simulink model "cantoni_combined_matrices_3pools_gates_hil_test"  (R2019b)
settings: Solver=FixedStepDiscrete  StartTime=0.0  StopTime=1000  FixedStep=1  RelTol=1e-3
values from neighbouring files (symbols this model uses):
  comb_contr = ss(Ac, Bc, Cc, Dc, h)    [cantoni_LMI.m]
  comb_plant_disc = c2d(comb_plant_cont,h,'zoh')    [cantoni_LMI.m]
  ddelay = [4 2 4 4 6]    [distributed_workspace.mat]
  Pd0 = c2d(P0, h, 'zoh')    [model_hil.m]
undefined symbols (not defined in the file or in its folder): Pd, Wd, Wis
settings Model: Creator=Jacob  LastModifiedBy=bas
settings SFSimCC: CustomCodeUndefinedFunction=UseInterfaceOnly

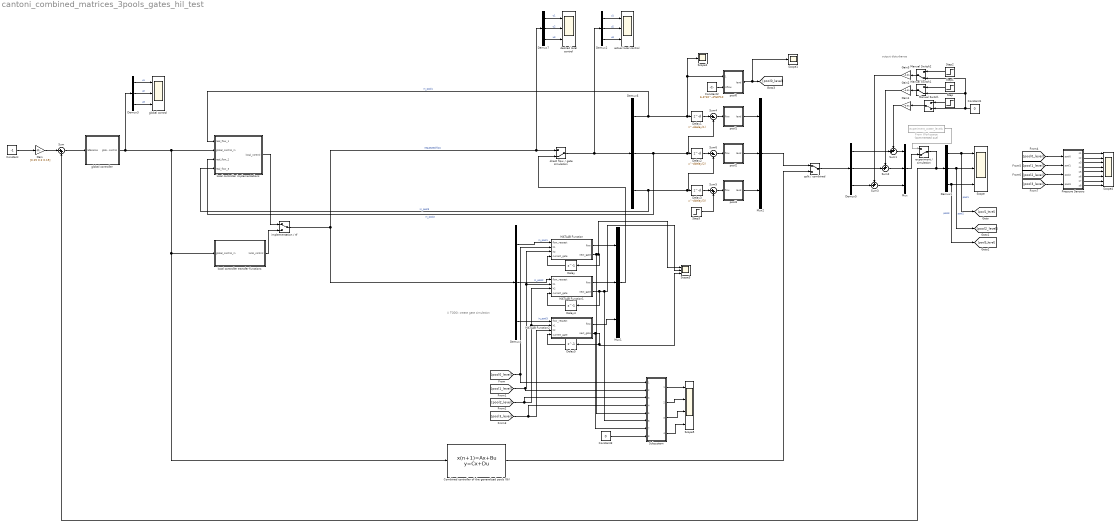
== system cantoni_combined_matrices_3pools_gates_hil_test ==
  note: // TODO: create gate simulation
  note: output disturbance
  Combined controller of the generalized pools (Gi) : DiscreteStateSpace  A=comb_plant_disc.A  B=comb_plant_disc.B  C=comb_plant_disc.C  D=comb_plant_disc.D  SampleTime=-1
  Constant : Constant  Value=-1
  Constant1 : Constant  Value=0
  Constant2 : Constant  Value=6.4*10^-4*60*10
  Constant3 : Constant  Value=0
  Delay : Delay  DelayLength=1
  Delay1 : Delay  DelayLength=ddelay(1)
  Delay2 : Delay  DelayLength=ddelay(2)
  Delay3 : Delay  DelayLength=ddelay(3)
  Delay4 : Delay  DelayLength=1
  Delay5 : Delay  DelayLength=1
  Demux{1..7} (7 alike) : Demux  Outputs=3
  From Workspace : FromWorkspace  Commented=on  VariableName=experiment_water_levels
  Gain : Gain  Gain=[0.25 0.2 0.15]
  Gain1 : Gain  Gain=-0.01
  Gain2 : Gain  Gain=-0.01
  Gain3 : Gain  Gain=-0.01
  MATLAB Function : MATLAB Function  TreatAsAtomicUnit=on
  MATLAB Function1 : MATLAB Function  TreatAsAtomicUnit=on
  MATLAB Function2 : MATLAB Function  TreatAsAtomicUnit=on
  Manual Switch : ManualSwitch  CurrentSetting=0
  Manual Switch1 : ManualSwitch  CurrentSetting=0
  Manual Switch2 : ManualSwitch  CurrentSetting=0
  Mux : Mux  Inputs=3
  Mux1 : Mux  Inputs=3
  Mux2 : Mux  Inputs=3
  Pressure Sensors : Subsystem
  Scope : Scope  NumInputPorts=3
  Scope1 : Scope
  Scope2 : Scope
  Scope3 : Scope  NumInputPorts=3
  Scope4 : Scope  NumInputPorts=8
  Scope5 : Scope  NumInputPorts=4
  Step : Step  Time=50  SampleTime=0
  Step1 : Step  Time=50  SampleTime=0
  Step2 : Step  Time=50  SampleTime=0
  Step3 : Step  Time=400  After=-3*10^-4*60*1  SampleTime=0
  Subsystem : Subsystem
  Sum : Sum  Inputs=|++
  Sum1 : Sum  Inputs=++|
  Sum2 : Sum  Inputs=++|
  Sum3 : Sum  Inputs=++|
  Sum4 : Sum  Inputs=|+-
  Sum5 : Sum  Inputs=|++
  Sum6 : Sum  Inputs=|+-
  actual local control : Scope  NumInputPorts=3
  desired local control : Scope  NumInputPorts=3
  direct flow / gate simulation : ManualSwitch  CurrentSetting=0
  experiment / simulation : ManualSwitch  CurrentSetting=0
  global control : Scope  NumInputPorts=3
  global controller : Subsystem
  implementation / tf : ManualSwitch
  local controller implementations : Subsystem
  local controller transfer functions : Subsystem
  pool0 : Subsystem
  pool1 : Subsystem
  pool2 : Subsystem
  pool3 : Subsystem
  split / combined : ManualSwitch
  wires:
  Constant/1 -> Gain/1
  Gain/1 -> Sum/1
  experiment / simulation/1 -> Sum/2, Demux1/1
  Demux1/1 -> Scope/1, [pool1_level]  "pool1"
  Demux1/2 -> [pool2_level], Scope/2  "pool2"
  Demux1/3 -> [pool3_level], Scope/3  "pool3"
  Step/1 -> Manual Switch/1
  Sum1/1 -> Mux/1
  Sum2/1 -> Mux/2
  Gain2/1 -> Sum2/1
  Step1/1 -> Manual Switch1/1
  Gain1/1 -> Sum1/1
  Manual Switch/1 -> Gain1/1
  Constant1/1 -> Manual Switch1/2, Manual Switch2/2, Manual Switch/2
  Manual Switch1/1 -> Gain2/1
  Sum3/1 -> Mux/3
  Manual Switch2/1 -> Gain3/1
  Step2/1 -> Manual Switch2/1
  Gain3/1 -> Sum3/1
  Demux3/3 -> global control/3  "u3"
  Demux3/2 -> global control/2  "u2"
  Demux3/1 -> global control/1  "u1"
  Demux5/1 -> Sum1/2
  Demux5/2 -> Sum2/2
  Demux5/3 -> Sum3/2
  split / combined/1 -> Demux5/1
  Mux2/1 -> split / combined/1
  Combined controller of the generalized pools (Gi)/1 -> split / combined/2
  Delay1/1 -> Sum4/1
  Delay2/1 -> Sum6/1
  Demux6/1 -> Scope2/1, pool0/1(outflow), Delay1/1, local controller implementations/1(real_flow_1)  "in_pool1"
  Demux6/2 -> Sum4/2, Delay2/1, local controller implementations/3(real_flow_2)  "in_pool2"
  Demux6/3 -> Sum6/2, Delay3/1, local controller implementations/4(real_flow_3)  "in_pool3"
  implementation / tf/1 -> Demux4/1, Demux7/1, direct flow / gate simulation/1  "requested flow"
  local controller implementations/1(local_control) -> implementation / tf/1
  local controller transfer functions/1(local_control) -> implementation / tf/2
  Mux1/1 -> direct flow / gate simulation/2
  Sum4/1 -> pool1/1(flow)
  pool1/1(level) -> Mux2/1
  Sum6/1 -> pool2/1(flow)
  pool2/1(level) -> Mux2/2
  Delay3/1 -> Sum5/1
  pool3/1(level) -> Mux2/3
  global controller/1(global_control) -> local controller implementations/2(global_control_in), local controller transfer functions/1(global_control_in), Combined controller of the generalized pools (Gi)/1, Demux3/1
  Sum/1 -> global controller/1(reference)
  Demux2/3 -> actual local control/3  "u3"
  Demux2/1 -> actual local control/1  "u1"
  Demux2/2 -> actual local control/2  "u2"
  direct flow / gate simulation/1 -> Demux2/1, Demux6/1
  pool0/1(level) -> Scope1/1, [pool0_level]
  MATLAB Function/1(flow) -> Mux1/1
  Demux4/1 -> MATLAB Function/1(flow_request)  "in_pool1"
  Demux4/2 -> MATLAB Function1/1(flow_request)  "in_pool2"
  Demux4/3 -> MATLAB Function2/1(flow_request)  "in_pool3"
  MATLAB Function/2(next_gate) -> Subsystem/5(servo1), Scope3/1, Delay/1
  Delay/1 -> MATLAB Function/4(current_gate)
  [pool0_level] -> MATLAB Function/2(h1), Subsystem/1(pool0)
  [pool1_level] -> Subsystem/2(pool1), MATLAB Function1/2(h1), MATLAB Function/3(h2)
  Delay4/1 -> MATLAB Function1/4(current_gate)
  MATLAB Function1/2(next_gate) -> Subsystem/6(servo2), Scope3/2, Delay4/1
  MATLAB Function1/1(flow) -> Mux1/2
  Delay5/1 -> MATLAB Function2/4(current_gate)
  MATLAB Function2/2(next_gate) -> Subsystem/7(servo3), Scope3/3, Delay5/1
  MATLAB Function2/1(flow) -> Mux1/3
  [pool2_level] -> Subsystem/3(pool2), MATLAB Function2/2(h1), MATLAB Function1/3(h2)
  [pool3_level] -> Subsystem/4(pool3), MATLAB Function2/3(h2)
  Constant2/1 -> pool0/2(inflow)
  Sum5/1 -> pool3/1(flow)
  Step3/1 -> Sum5/2
  Mux/1 -> experiment / simulation/2
  From Workspace/1 -> experiment / simulation/1
  Demux7/3 -> desired local control/3  "u3"
  Demux7/2 -> desired local control/2  "u2"
  Demux7/1 -> desired local control/1  "u1"
  Pressure Sensors/1(s1) -> Scope4/1
  Pressure Sensors/2(s2) -> Scope4/2
  Pressure Sensors/3(s3) -> Scope4/3
  Pressure Sensors/4(s4) -> Scope4/4
  Pressure Sensors/5(s5) -> Scope4/5
  Pressure Sensors/6(s6) -> Scope4/6
  Pressure Sensors/7(s7) -> Scope4/7
  Pressure Sensors/8(s8) -> Scope4/8
  [pool0_level] -> Pressure Sensors/1(pool0)
  [pool1_level] -> Pressure Sensors/2(pool1)
  [pool2_level] -> Pressure Sensors/3(pool2)
  [pool3_level] -> Pressure Sensors/4(pool3)
  Constant3/1 -> Subsystem/8(servo4)
  Subsystem/1(flow0_1) -> Scope5/1
  Subsystem/2(flow1_2) -> Scope5/2
  Subsystem/3(flow2_3) -> Scope5/3
  Subsystem/4(flow3_4) -> Scope5/4

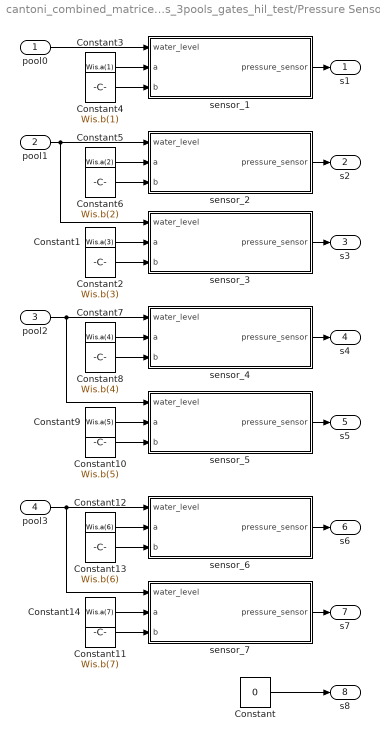
== system cantoni_combined_matrices_3pools_gates_hil_test/Pressure Sensors ==
  pool0 : Inport
  pool1 : Inport  Port=2
  pool2 : Inport  Port=3
  pool3 : Inport  Port=4
  Constant : Constant  Value=0
  Constant1 : Constant  Value=Wis.a(3)
  Constant10 : Constant  Value=Wis.b(5)
  Constant11 : Constant  Value=Wis.b(7)
  Constant12 : Constant  Value=Wis.a(6)
  Constant13 : Constant  Value=Wis.b(6)
  Constant14 : Constant  Value=Wis.a(7)
  Constant2 : Constant  Value=Wis.b(3)
  Constant3 : Constant  Value=Wis.a(1)
  Constant4 : Constant  Value=Wis.b(1)
  Constant5 : Constant  Value=Wis.a(2)
  Constant6 : Constant  Value=Wis.b(2)
  Constant7 : Constant  Value=Wis.a(4)
  Constant8 : Constant  Value=Wis.b(4)
  Constant9 : Constant  Value=Wis.a(5)
  sensor_1 : MATLAB Function  TreatAsAtomicUnit=on
  sensor_2 : MATLAB Function  TreatAsAtomicUnit=on
  sensor_3 : MATLAB Function  TreatAsAtomicUnit=on
  sensor_4 : MATLAB Function  TreatAsAtomicUnit=on
  sensor_5 : MATLAB Function  TreatAsAtomicUnit=on
  sensor_6 : MATLAB Function  TreatAsAtomicUnit=on
  sensor_7 : MATLAB Function  TreatAsAtomicUnit=on
  s1 : Outport
  s2 : Outport  Port=2
  s3 : Outport  Port=3
  s4 : Outport  Port=4
  s5 : Outport  Port=5
  s6 : Outport  Port=6
  s7 : Outport  Port=7
  s8 : Outport  Port=8
  wires:
  sensor_1/1(pressure_sensor) -> s1/1
  Constant5/1 -> sensor_2/2(a)
  Constant3/1 -> sensor_1/2(a)
  Constant4/1 -> sensor_1/3(b)
  Constant6/1 -> sensor_2/3(b)
  sensor_2/1(pressure_sensor) -> s2/1
  pool0/1 -> sensor_1/1(water_level)
  Constant1/1 -> sensor_3/2(a)
  Constant2/1 -> sensor_3/3(b)
  sensor_3/1(pressure_sensor) -> s3/1
  sensor_4/1(pressure_sensor) -> s4/1
  Constant7/1 -> sensor_4/2(a)
  Constant8/1 -> sensor_4/3(b)
  Constant10/1 -> sensor_5/3(b)
  Constant9/1 -> sensor_5/2(a)
  pool2/1 -> sensor_5/1(water_level), sensor_4/1(water_level)
  sensor_5/1(pressure_sensor) -> s5/1
  Constant12/1 -> sensor_6/2(a)
  pool3/1 -> sensor_7/1(water_level), sensor_6/1(water_level)
  sensor_6/1(pressure_sensor) -> s6/1
  Constant13/1 -> sensor_6/3(b)
  Constant11/1 -> sensor_7/3(b)
  Constant14/1 -> sensor_7/2(a)
  sensor_7/1(pressure_sensor) -> s7/1
  Constant/1 -> s8/1
  pool1/1 -> sensor_3/1(water_level), sensor_2/1(water_level)

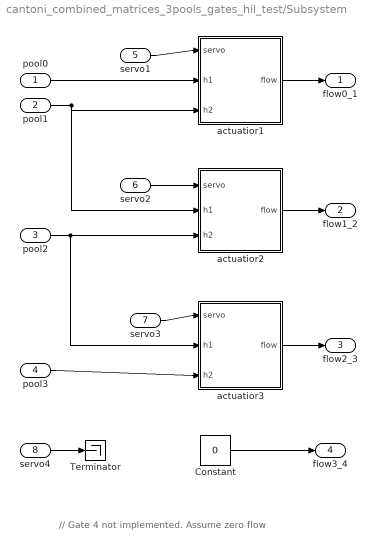
== system cantoni_combined_matrices_3pools_gates_hil_test/Subsystem ==
  note: // Gate 4 not implemented. Assume zero flow
  pool0 : Inport
  pool1 : Inport  Port=2
  pool2 : Inport  Port=3
  pool3 : Inport  Port=4
  servo1 : Inport  Port=5
  servo2 : Inport  Port=6
  servo3 : Inport  Port=7
  servo4 : Inport  Port=8
  Constant : Constant  Value=0
  Terminator : Terminator
  actuatior1 : MATLAB Function  TreatAsAtomicUnit=on
  actuatior2 : MATLAB Function  TreatAsAtomicUnit=on
  actuatior3 : MATLAB Function  TreatAsAtomicUnit=on
  flow0_1 : Outport
  flow1_2 : Outport  Port=2
  flow2_3 : Outport  Port=3
  flow3_4 : Outport  Port=4
  wires:
  pool1/1 -> actuatior2/2(h1), actuatior1/3(h2)
  servo2/1 -> actuatior2/1(servo)
  pool2/1 -> actuatior3/2(h1), actuatior2/3(h2)
  actuatior1/1(flow) -> flow0_1/1
  servo1/1 -> actuatior1/1(servo)
  servo3/1 -> actuatior3/1(servo)
  pool0/1 -> actuatior1/2(h1)
  actuatior2/1(flow) -> flow1_2/1
  pool3/1 -> actuatior3/3(h2)
  actuatior3/1(flow) -> flow2_3/1
  servo4/1 -> Terminator/1
  Constant/1 -> flow3_4/1

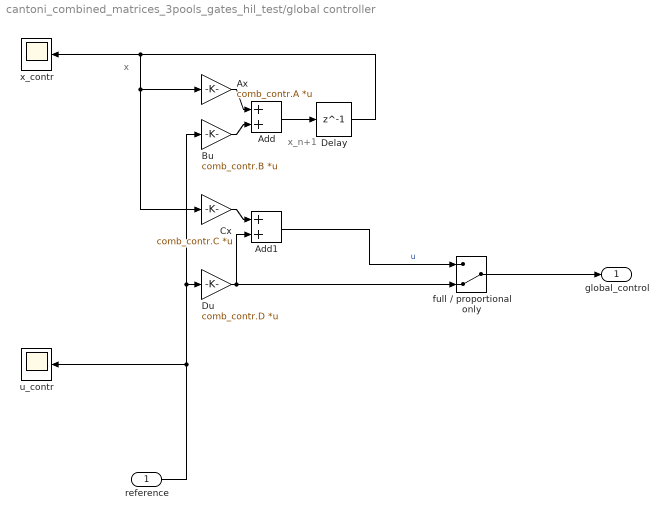
== system cantoni_combined_matrices_3pools_gates_hil_test/global controller ==
  note: x
  note: x_n+1
  reference : Inport
  Add : Sum
  Add1 : Sum
  Ax : Gain  Gain=comb_contr.A  Multiplication=Matrix(K*u)
  Bu : Gain  Gain=comb_contr.B  Multiplication=Matrix(K*u)
  Cx : Gain  Gain=comb_contr.C  Multiplication=Matrix(K*u)
  Delay : Delay  DelayLength=1  InitialCondition=[0;0;0;0;0;0;0;0;0;0;0;0;0;0;0]
  Du : Gain  Gain=comb_contr.D  Multiplication=Matrix(K*u)
  full / proportional only : ManualSwitch  CurrentSetting=0
  u_contr : Scope
  x_contr : Scope
  global_control : Outport
  wires:
  Bu/1 -> Add/2
  Cx/1 -> Add1/1
  Add/1 -> Delay/1
  Add1/1 -> full / proportional only/1  "u"
  Ax/1 -> Add/1
  Du/1 -> Add1/2, full / proportional only/2
  full / proportional only/1 -> global_control/1
  Delay/1 -> x_contr/1, Cx/1, Ax/1
  reference/1 -> Bu/1, Du/1, u_contr/1

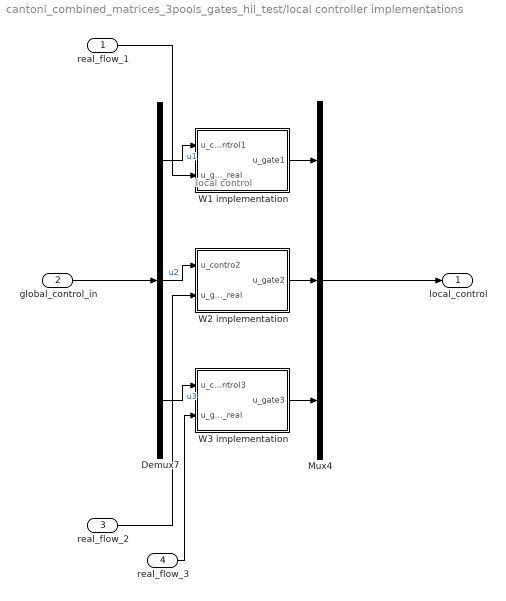
== system cantoni_combined_matrices_3pools_gates_hil_test/local controller implementations ==
  note: local control
  real_flow_1 : Inport
  global_control_in : Inport  Port=2
  real_flow_2 : Inport  Port=3
  real_flow_3 : Inport  Port=4
  Demux7 : Demux  Outputs=3
  Mux4 : Mux  Inputs=3
  W1 implementation : Subsystem
  W2 implementation : Subsystem
  W3 implementation : Subsystem
  local_control : Outport
  wires:
  Demux7/1 -> W1 implementation/1(u_control1)  "u1"
  W1 implementation/1(u_gate1) -> Mux4/1
  Demux7/3 -> W3 implementation/1(u_control3)  "u3"
  real_flow_3/1 -> W3 implementation/2(u_gate3_real)
  real_flow_2/1 -> W2 implementation/2(u_gate2_real)
  Demux7/2 -> W2 implementation/1(u_contro2)  "u2"
  global_control_in/1 -> Demux7/1
  Mux4/1 -> local_control/1
  W3 implementation/1(u_gate3) -> Mux4/3
  real_flow_1/1 -> W1 implementation/2(u_gate1_real)
  W2 implementation/1(u_gate2) -> Mux4/2

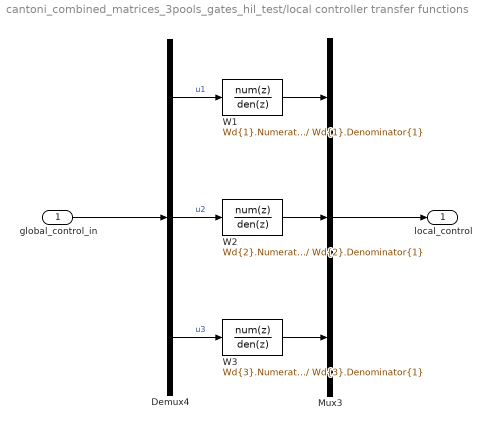
== system cantoni_combined_matrices_3pools_gates_hil_test/local controller transfer functions ==
  global_control_in : Inport
  Demux4 : Demux  Outputs=3
  Mux3 : Mux  Inputs=3
  W1 : DiscreteTransferFcn  Numerator=Wd{1}.Numerator{1}  Denominator=Wd{1}.Denominator{1}
  W2 : DiscreteTransferFcn  Numerator=Wd{2}.Numerator{1}  Denominator=Wd{2}.Denominator{1}
  W3 : DiscreteTransferFcn  Numerator=Wd{3}.Numerator{1}  Denominator=Wd{3}.Denominator{1}
  local_control : Outport
  wires:
  Mux3/1 -> local_control/1
  global_control_in/1 -> Demux4/1
  Demux4/3 -> W3/1  "u3"
  W3/1 -> Mux3/3
  Demux4/2 -> W2/1  "u2"
  W2/1 -> Mux3/2
  W1/1 -> Mux3/1
  Demux4/1 -> W1/1  "u1"

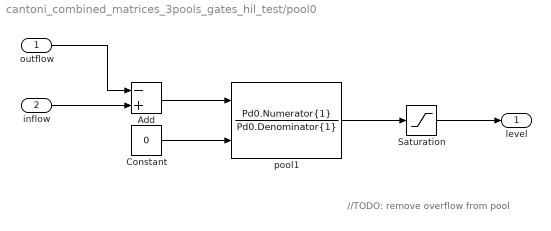
== system cantoni_combined_matrices_3pools_gates_hil_test/pool0 ==
  note: //TODO: remove overflow from pool
  outflow : Inport
  inflow : Inport  Port=2
  Add : Sum  Inputs=-+
  Constant : Constant  Value=0
  Saturation : Saturate  UpperLimit=0.6
  pool1 : DiscreteTransferFcn  Numerator=Pd0.Numerator{1}  Denominator=Pd0.Denominator{1}  InitialStatesSource=Input port
      settings: InputPortMap=u0,p5
  level : Outport
  wires:
  pool1/1 -> Saturation/1
  outflow/1 -> Add/1
  inflow/1 -> Add/2
  Add/1 -> pool1/1
  Constant/1 -> pool1/2
  Saturation/1 -> level/1

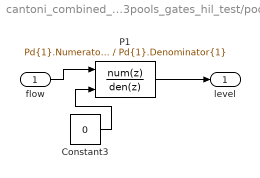
== system cantoni_combined_matrices_3pools_gates_hil_test/pool1 ==
  flow : Inport
  Constant3 : Constant  Value=0  SampleTime=-1
  P1 : DiscreteTransferFcn  Numerator=Pd{1}.Numerator{1}  Denominator=Pd{1}.Denominator{1}  InitialStatesSource=Input port
      settings: InputPortMap=u0,p5
  level : Outport
  wires:
  flow/1 -> P1/1
  P1/1 -> level/1
  Constant3/1 -> P1/2

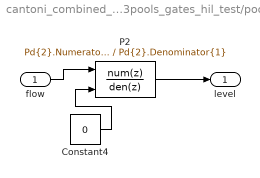
== system cantoni_combined_matrices_3pools_gates_hil_test/pool2 ==
  flow : Inport
  Constant4 : Constant  Value=0
  P2 : DiscreteTransferFcn  Numerator=Pd{2}.Numerator{1}  Denominator=Pd{2}.Denominator{1}  InitialStatesSource=Input port
      settings: InputPortMap=u0,p5
  level : Outport
  wires:
  flow/1 -> P2/1
  P2/1 -> level/1
  Constant4/1 -> P2/2

== system cantoni_combined_matrices_3pools_gates_hil_test/pool3 ==
  flow : Inport
  Constant5 : Constant  Value=0
  P3 : DiscreteTransferFcn  Numerator=Pd{3}.Numerator{1}  Denominator=Pd{3}.Denominator{1}  InitialStatesSource=Input port
      settings: InputPortMap=u0,p5
  level : Outport
  wires:
  P3/1 -> level/1
  flow/1 -> P3/1
  Constant5/1 -> P3/2

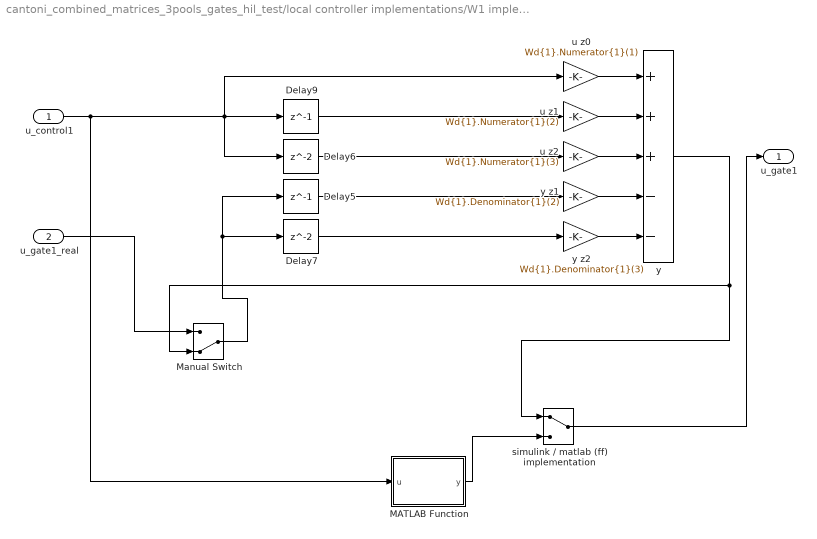
== system cantoni_combined_matrices_3pools_gates_hil_test/local controller implementations/W1 implementation ==
  u_control1 : Inport
  u_gate1_real : Inport  Port=2
  Delay5 : Delay  DelayLength=1
  Delay6 : Delay
  Delay7 : Delay
  Delay9 : Delay  DelayLength=1
  MATLAB Function : MATLAB Function  TreatAsAtomicUnit=on
  Manual Switch : ManualSwitch  CurrentSetting=0
  simulink / matlab (ff) implementation : ManualSwitch
  u z0 : Gain  Gain=Wd{1}.Numerator{1}(1)
  u z1 : Gain  Gain=Wd{1}.Numerator{1}(2)
  u z2 : Gain  Gain=Wd{1}.Numerator{1}(3)
  y : Sum  Inputs=+++--
  y z1 : Gain  Gain=Wd{1}.Denominator{1}(2)
  y z2 : Gain  Gain=Wd{1}.Denominator{1}(3)
  u_gate1 : Outport
  wires:
  y z2/1 -> y/5
  Delay6/1 -> u z2/1
  y z1/1 -> y/4
  Delay7/1 -> y z2/1
  u z1/1 -> y/2
  u z2/1 -> y/3
  y/1 -> simulink / matlab (ff) implementation/1, Manual Switch/2
  Delay5/1 -> y z1/1
  u_control1/1 -> MATLAB Function/1(u), Delay6/1, u z0/1, Delay9/1
  u z0/1 -> y/1
  Delay9/1 -> u z1/1
  Manual Switch/1 -> Delay5/1, Delay7/1
  u_gate1_real/1 -> Manual Switch/1
  MATLAB Function/1(y) -> simulink / matlab (ff) implementation/2
  simulink / matlab (ff) implementation/1 -> u_gate1/1

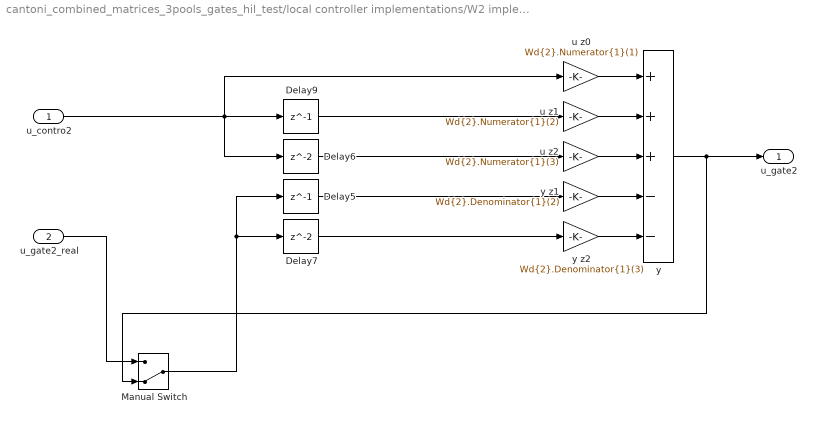
== system cantoni_combined_matrices_3pools_gates_hil_test/local controller implementations/W2 implementation ==
  u_contro2 : Inport
  u_gate2_real : Inport  Port=2
  Delay5 : Delay  DelayLength=1
  Delay6 : Delay
  Delay7 : Delay
  Delay9 : Delay  DelayLength=1
  Manual Switch : ManualSwitch  CurrentSetting=0
  u z0 : Gain  Gain=Wd{2}.Numerator{1}(1)
  u z1 : Gain  Gain=Wd{2}.Numerator{1}(2)
  u z2 : Gain  Gain=Wd{2}.Numerator{1}(3)
  y : Sum  Inputs=+++--
  y z1 : Gain  Gain=Wd{2}.Denominator{1}(2)
  y z2 : Gain  Gain=Wd{2}.Denominator{1}(3)
  u_gate2 : Outport
  wires:
  y z2/1 -> y/5
  Delay6/1 -> u z2/1
  y z1/1 -> y/4
  Delay7/1 -> y z2/1
  u z1/1 -> y/2
  u z2/1 -> y/3
  y/1 -> Manual Switch/2, u_gate2/1
  Delay5/1 -> y z1/1
  u_contro2/1 -> Delay6/1, u z0/1, Delay9/1
  u z0/1 -> y/1
  Delay9/1 -> u z1/1
  Manual Switch/1 -> Delay5/1, Delay7/1
  u_gate2_real/1 -> Manual Switch/1

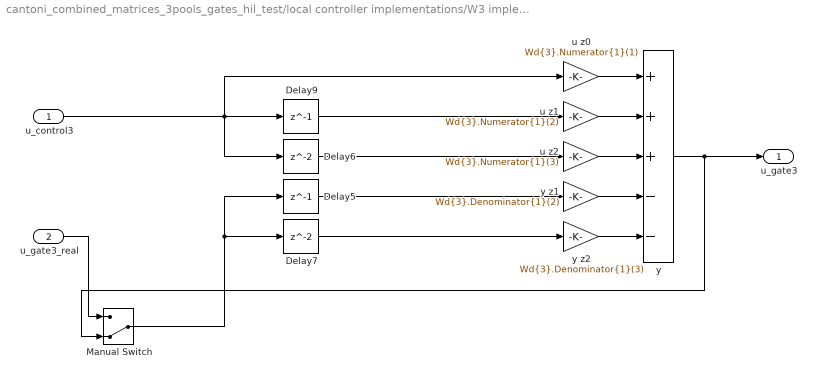
== system cantoni_combined_matrices_3pools_gates_hil_test/local controller implementations/W3 implementation ==
  u_control3 : Inport
  u_gate3_real : Inport  Port=2
  Delay5 : Delay  DelayLength=1
  Delay6 : Delay
  Delay7 : Delay
  Delay9 : Delay  DelayLength=1
  Manual Switch : ManualSwitch  CurrentSetting=0
  u z0 : Gain  Gain=Wd{3}.Numerator{1}(1)
  u z1 : Gain  Gain=Wd{3}.Numerator{1}(2)
  u z2 : Gain  Gain=Wd{3}.Numerator{1}(3)
  y : Sum  Inputs=+++--
  y z1 : Gain  Gain=Wd{3}.Denominator{1}(2)
  y z2 : Gain  Gain=Wd{3}.Denominator{1}(3)
  u_gate3 : Outport
  wires:
  y z2/1 -> y/5
  Delay6/1 -> u z2/1
  y z1/1 -> y/4
  Delay7/1 -> y z2/1
  u z1/1 -> y/2
  u z2/1 -> y/3
  y/1 -> Manual Switch/2, u_gate3/1
  Delay5/1 -> y z1/1
  u_control3/1 -> Delay6/1, u z0/1, Delay9/1
  u z0/1 -> y/1
  Delay9/1 -> u z1/1
  Manual Switch/1 -> Delay5/1, Delay7/1
  u_gate3_real/1 -> Manual Switch/1

== matlab function cantoni_combined_matrices_3pools_gates_hil_test/MATLAB Function1 ==
  data: flow_request input; flow output; h1 input; h2 input; current_gate input; next_gate output
function [flow, next_gate] = fcn(flow_request, h1, h2, current_gate)

[flow, next_gate] = gate_simulation(flow_request, h1, h2, current_gate);

== matlab function cantoni_combined_matrices_3pools_gates_hil_test/MATLAB Function ==
  data: flow_request input; flow output; h1 input; h2 input; current_gate input; next_gate output
function [flow, next_gate] = fcn(flow_request, h1, h2, current_gate)

[flow, next_gate] = gate_simulation(flow_request, h1, h2, current_gate);

== matlab function cantoni_combined_matrices_3pools_gates_hil_test/MATLAB Function2 ==
  data: flow_request input; flow output; h1 input; h2 input; current_gate input; next_gate output
function [flow, next_gate] = fcn(flow_request, h1, h2, current_gate)

[flow, next_gate] = gate_simulation(flow_request, h1, h2, current_gate);

== matlab function cantoni_combined_matrices_3pools_gates_hil_test/local controller implementations/W1 implementation/MATLAB Function ==
  data: u input; y output
function y = fcn(u)

persistent y_z1;
persistent y_z0;
persistent u_z1;
persistent u_z0;

if isempty(y_z1)
 y_z1 = 0;
 y_z0 = 0;
 u_z1 = 0;
 u_z0 = 0;
end


ku0 = 1.539744e-01;
ku1 = 2.564103e-04;
ku2 = -1.537179e-01;
ky1 = -1.846154e+00;
ky2 = 8.461538e-01;
    %// calculate y
y = ku0 * u + ku1 * u_z0 + ku2 * u_z1 - ky1 * y_z0 - ky2 * y_z1;

    %// update delays
    y_z1 = y_z0;
    y_z0 = y; %// not useful anymore due to ant-wind-up scheme
    u_z1 = u_z0;
    u_z0 = u; %// not useful anymore due to ant-wind-up scheme



% static double ku0[NUM_ACTUATORS] = {1.539744e-01, 2.309615e-01, 1.539744e-01};
% static double ku1[NUM_ACTUATORS] = {2.564103e-04, 3.846154e-04, 2.564103e-04};
% static double ku2[NUM_ACTUATORS] = {-1.537179e-01, -2.305769e-01, -1.537179e-01};
% static double ky1[NUM_ACTUATORS] = {-1.846154e+00, -1.846154e+00, -1.846154e+00};
% static double ky2[NUM_ACTUATORS] = {8.461538e-01, 8.461538e-01, 8.461538e-01};

== matlab function cantoni_combined_matrices_3pools_gates_hil_test/Pressure Sensors/sensor_1 ==
  data: water_level input; pressure_sensor output; a input; b input
function pressure_sensor = fcn(water_level, a, b)

pressure_sensor = m2pressure(water_level, a, b);

== matlab function cantoni_combined_matrices_3pools_gates_hil_test/Pressure Sensors/sensor_2 ==
  data: water_level input; pressure_sensor output; a input; b input
function pressure_sensor = fcn(water_level, a, b)

pressure_sensor = m2pressure(water_level, a, b);

== matlab function cantoni_combined_matrices_3pools_gates_hil_test/Pressure Sensors/sensor_3 ==
  data: water_level input; pressure_sensor output; a input; b input
function pressure_sensor = fcn(water_level, a, b)

pressure_sensor = m2pressure(water_level, a, b);

== matlab function cantoni_combined_matrices_3pools_gates_hil_test/Pressure Sensors/sensor_4 ==
  data: water_level input; pressure_sensor output; a input; b input
function pressure_sensor = fcn(water_level, a, b)

pressure_sensor = m2pressure(water_level, a, b);

== matlab function cantoni_combined_matrices_3pools_gates_hil_test/Pressure Sensors/sensor_5 ==
  data: water_level input; pressure_sensor output; a input; b input
function pressure_sensor = fcn(water_level, a, b)

pressure_sensor = m2pressure(water_level, a, b);

== matlab function cantoni_combined_matrices_3pools_gates_hil_test/Pressure Sensors/sensor_6 ==
  data: water_level input; pressure_sensor output; a input; b input
function pressure_sensor = fcn(water_level, a, b)

pressure_sensor = m2pressure(water_level, a, b);

== matlab function cantoni_combined_matrices_3pools_gates_hil_test/Pressure Sensors/sensor_7 ==
  data: water_level input; pressure_sensor output; a input; b input
function pressure_sensor = fcn(water_level, a, b)

pressure_sensor = m2pressure(water_level, a, b);

== matlab function cantoni_combined_matrices_3pools_gates_hil_test/Subsystem/actuatior1 ==
  data: servo input; flow output; h1 input; h2 input
function flow = fcn(servo, h1, h2)

flow = gate2flow(servo, h1, h2);

== matlab function cantoni_combined_matrices_3pools_gates_hil_test/Subsystem/actuatior2 ==
  data: servo input; flow output; h1 input; h2 input
function flow = fcn(servo, h1, h2)

flow = gate2flow(servo, h1, h2);

== matlab function cantoni_combined_matrices_3pools_gates_hil_test/Subsystem/actuatior3 ==
  data: servo input; flow output; h1 input; h2 input
function flow = fcn(servo, h1, h2)

flow = gate2flow(servo, h1, h2);
